simulink model "DYNctl_ver4_etud_obfusc"  (R2019a)
settings: Solver=ode45  StartTime=0.0  StopTime=tfin  FixedStep=0.001  RelTol=1e-09  EnableMultiTasking=on
values from neighbouring files (symbols this model uses):
  ae0 = 1.346257119209160    (= 1.34625711921)    [bancEssaiConstantes.m]
  ae1 = 3.490773781399032e+02    (= 349.07737814)    [bancEssaiConstantes.m]
  ae2 = 1.450384791542791e+03    (= 1450.38479154)    [bancEssaiConstantes.m]
  ae3 = 7.033442113266084e+05    (= 703344.211327)    [bancEssaiConstantes.m]
  as0 = 0.040978814093345    (= 0.0409788140933)    [bancEssaiConstantes.m]
  as1 = 10.275913216141866    (= 10.2759132161)    [bancEssaiConstantes.m]
  as2 = -4.149770657537117e+02    (= -414.977065754)    [bancEssaiConstantes.m]
  as3 = 5.763371762601417e+03    (= 5763.3717626)    [bancEssaiConstantes.m]
  be1 = 13.029359254409743    (= 13.0293592544)    [bancEssaiConstantes.m]
  g = 9.81    [bancEssaiConstantes.m]
  Jx = 1169e-06    (= 0.001169)    [bancEssaiConstantes.m]
  LL = .115    (= 0.115)    [bancEssaiConstantes.m]
  mP = 425e-03    (= 0.425)    [bancEssaiConstantes.m]
  mS = 0.0080    (= 0.008)    [bancEssaiConstantes.m]
  offset = 7.563899999998686    (= 7.5639)    [bancEssaiConstantes.m]
  RR = 3.6    [bancEssaiConstantes.m]
  Vmax = 16.0    (= 16)    [bancEssaiConstantes.m]
  XA = +rABC    (= 0.0952)    [bancEssaiConstantes.m]
  XB = -rABC*sind(30)    [bancEssaiConstantes.m]
  XC = -rABC*sind(30)    [bancEssaiConstantes.m]
  XD = +rDEF*sind(30)    [bancEssaiConstantes.m]
  XE = -rDEF    (= -0.08)    [bancEssaiConstantes.m]
  XF = +rDEF*sind(30)    [bancEssaiConstantes.m]
  YA = 0.0    (= 0)    [bancEssaiConstantes.m]
  YB = +rABC*cosd(30)    [bancEssaiConstantes.m]
  YC = -rABC*cosd(30)    [bancEssaiConstantes.m]
  YD = +rDEF*cosd(30)    [bancEssaiConstantes.m]
  YE = 0.0    (= 0)    [bancEssaiConstantes.m]
  YF = -rDEF*cosd(30)    [bancEssaiConstantes.m]
settings Model: Creator=delafontaine  LastModifiedBy=gaul2525
settings SolverCC: AlgebraicLoopSolver=LineSearch
settings DataIOCC: LimitDataPoints=on  SaveFormat=Array  SignalLoggingSaveFormat=ModelDataLogs  ReturnWorkspaceOutputs=off
settings OptimizationCC: LifeSpan=inf
settings DebuggingCC: UnderspecifiedInitializationDetection=Classic  MergeDetectMultiDrivingBlocksExec=none  MultiTaskDSMMsg=warning  MultiTaskCondExecSysMsg=none  SFUnexpectedBacktrackingDiag=warning  SFNoUnconditionalDefaultTransitionDiag=warning  SFExecutionAtInitializationDiag=none  UnderSpecifiedDimensionMsg=warning  ArithmeticOperatorsInVariantConditions=warning
settings HardwareCC: ProdBitPerPointer=32  ProdBitPerSizeT=32  ProdBitPerPtrDiffT=32  ProdLargestAtomicFloat=None  ProdIntDivRoundTo=Undefined  ProdEndianess=Unspecified  ProdWordSize=32  ProdHWDeviceType=32-bit Generic
settings ModelReferenceCC: PropagateSignalLabelsOutOfModel=off
settings SFSimCC: SimUseLocalCustomCode=off
settings RTWCC: RTWUseLocalCustomCode=off
settings CodeAppCC: StateflowObjectComments=on
settings GRTTargetCC: TargetLangStandard=C89/C90 (ANSI)  GeneratePreprocessorConditionals=Disable all
settings ConfigComp: CovMetricSettings=dw  CovHtmlReporting=on  CovSaveCumulativeToWorkspaceVar=on  CovSaveSingleToWorkspaceVar=on  CovExternalEMLEnable=off  CovSFcnEnable=off

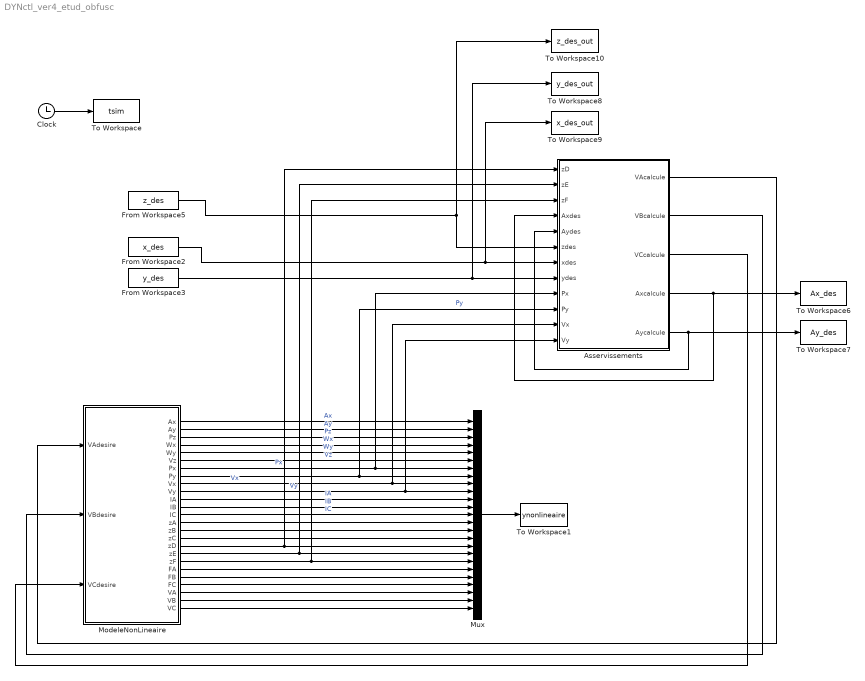
== system DYNctl_ver4_etud_obfusc ==
  Asservissements : Subsystem
      mask help: Simulink:masks:GenSFuncDesc_MD
      mask Help: eval('feval(''rtwprivate'',''rtwhelpview'',''rtw_sfcn_block'')');
  Clock : Clock
  From Workspace2 : FromWorkspace  VariableName=x_des  SampleTime=0  Interpolate=off  OutputAfterFinalValue=Holding final value
  From Workspace3 : FromWorkspace  VariableName=y_des  SampleTime=0  Interpolate=off  OutputAfterFinalValue=Holding final value
  From Workspace5 : FromWorkspace  VariableName=z_des  SampleTime=0  Interpolate=off  OutputAfterFinalValue=Holding final value
  ModeleNonLineaire : Subsystem
      mask help: Simulink:masks:GenSFuncDesc_MD
      mask Help: eval('feval(''rtwprivate'',''rtwhelpview'',''rtw_sfcn_block'')');
  Mux : Mux  Inputs=25
  To Workspace : ToWorkspace  VariableName=tsim  SampleTime=-1
  To Workspace1 : ToWorkspace  VariableName=ynonlineaire  SampleTime=-1
  To Workspace10 : ToWorkspace  VariableName=z_des_out  SampleTime=-1
  To Workspace6 : ToWorkspace  VariableName=Ax_des  SampleTime=-1
  To Workspace7 : ToWorkspace  VariableName=Ay_des  SampleTime=-1
  To Workspace8 : ToWorkspace  VariableName=y_des_out  SampleTime=-1
  To Workspace9 : ToWorkspace  VariableName=x_des_out  SampleTime=-1
  wires:
  Mux/1 -> To Workspace1/1
  Clock/1 -> To Workspace/1
  From Workspace5/1 -> Asservissements/6(zdes), To Workspace10/1
  ModeleNonLineaire/1(Ax) -> Mux/1  "Ax"
  ModeleNonLineaire/2(Ay) -> Mux/2  "Ay"
  ModeleNonLineaire/3(Pz) -> Mux/3  "Pz"
  ModeleNonLineaire/4(Wx) -> Mux/4  "Wx"
  ModeleNonLineaire/5(Wy) -> Mux/5  "Wy"
  ModeleNonLineaire/6(Vz) -> Mux/6  "Vz"
  ModeleNonLineaire/7(Px) -> Asservissements/9(Px), Mux/7  "Px"
  ModeleNonLineaire/8(Py) -> Asservissements/10(Py), Mux/8  "Py"
  ModeleNonLineaire/9(Vx) -> Asservissements/11(Vx), Mux/9  "Vx"
  ModeleNonLineaire/10(Vy) -> Asservissements/12(Vy), Mux/10  "Vy"
  ModeleNonLineaire/11(IA) -> Mux/11  "IA"
  ModeleNonLineaire/12(IB) -> Mux/12  "IB"
  ModeleNonLineaire/13(IC) -> Mux/13  "IC"
  From Workspace3/1 -> Asservissements/8(ydes), To Workspace8/1
  From Workspace2/1 -> Asservissements/7(xdes), To Workspace9/1
  ModeleNonLineaire/20(FA) -> Mux/20
  ModeleNonLineaire/21(FB) -> Mux/21
  ModeleNonLineaire/22(FC) -> Mux/22
  ModeleNonLineaire/23(VA) -> Mux/23
  ModeleNonLineaire/24(VB) -> Mux/24
  ModeleNonLineaire/25(VC) -> Mux/25
  ModeleNonLineaire/17(zD) -> Asservissements/1(zD), Mux/17
  ModeleNonLineaire/18(zE) -> Asservissements/2(zE), Mux/18
  ModeleNonLineaire/19(zF) -> Asservissements/3(zF), Mux/19
  ModeleNonLineaire/14(zA) -> Mux/14
  ModeleNonLineaire/15(zB) -> Mux/15
  ModeleNonLineaire/16(zC) -> Mux/16
  Asservissements/4(Axcalcule) -> Asservissements/4(Axdes), To Workspace6/1
  Asservissements/5(Aycalcule) -> Asservissements/5(Aydes), To Workspace7/1
  Asservissements/1(VAcalcule) -> ModeleNonLineaire/1(VAdesire)
  Asservissements/2(VBcalcule) -> ModeleNonLineaire/2(VBdesire)
  Asservissements/3(VCcalcule) -> ModeleNonLineaire/3(VCdesire)

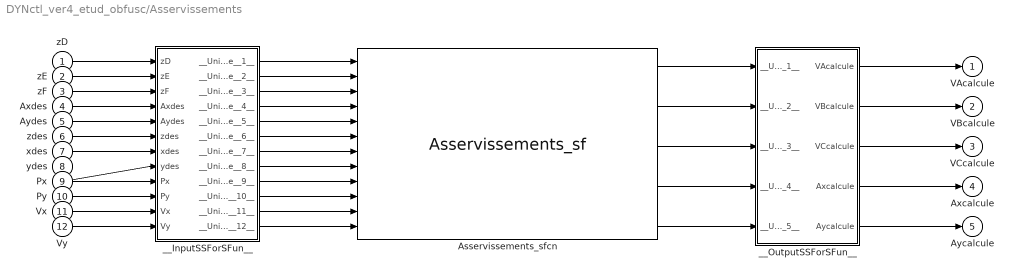
== system DYNctl_ver4_etud_obfusc/Asservissements ==
  zD : Inport
  zE : Inport  Port=2
  zF : Inport  Port=3
  Axdes : Inport  Port=4
  Aydes : Inport  Port=5
  zdes : Inport  Port=6
  xdes : Inport  Port=7
  ydes : Inport  Port=8
  Px : Inport  Port=9
  Py : Inport  Port=10
  Vx : Inport  Port=11
  Vy : Inport  Port=12
  Asservissements_sfcn : S-Function  FunctionName=Asservissements_sf  SFunctionModules=""  SFunctionDeploymentMode=off  EnableBusSupport=off  mask{rtw_sf_name=Asservissements_sf, showVar=off}
      mask prompts: rtw_sf_name "Simulink:masks:GenSFuncName_MP"; showVar "Simulink:masks:GenSFuncShowModuleList_MP"
      mask help: Simulink:masks:GenSFuncDesc_MD
      mask init:
      | displist = '';
      | if ~strcmp(get_param(gcb, 'FunctionName'), rtw_sf_name);
      |   set_param(gcb, 'FunctionName', rtw_sf_name);
      | end
      | % Check if we are generating code
      | rtw_mode = false;
      | if strcmpi(get_param(bdroot(gcb),'SimulationStatus'),'Initializing')
      | 	rtw_mode = strcmpi(get_param(bdroot(gcb),'BuildingRTWCode'),'on') && ...
      | 		~strcmpi(get_param(bdroot(gcb),'TargetStyle'),'SimulationTarget');
      | end
      | if showVar || rtw_mode
      | 	if exist('rtwsfunc') == 2 | exist('rtwsfunc') == 6
      | 		tmplist = rtwsfunc(rtw_sf_name,gcb);
      | 		tmplist = DAStudio.message('Simulink:masks:GenSFuncListOfModules_IC', tmplist);
      | 	elseif showVar
      | 		tmplist1 = DAStudio.message('Simulink:masks:GenSFuncListOfModules_IC', '');
      |         tmplist2 = DAStudio.message('Simulink:masks:GenSFuncNotLicensed_IC');
      |         tmplist = [tmplist1 tmplist2];
      |  	end
      | end
      | if showVar
      |   displist = tmplist;
      | end
      settings: CopyFcn=|
      | if ~strcmp(get_param(gcb,'Linkstatus'),'none') && ...
      | ~strcmp(get_param(gcb,'Linkstatus'),'implicit')
      |   set_param(gcb,'LinkStatus','none');
      | end
      mask Help: eval('feval(''rtwprivate'',''rtwhelpview'',''rtw_sfcn_block'')');
      mask Display:
      | port_label('input',1,'zD');
      | port_label('input',2,'zE');
      | port_label('input',3,'zF');
      | port_label('input',4,'Axdes');
      | port_label('input',5,'Aydes');
      | port_label('input',6,'zdes');
      | port_label('input',7,'xdes');
      | port_label('input',8,'ydes');
      | port_label('input',9,'Px');
      | port_label('input',10,'Py');
      | port_label('input',11,'Vx');
      | port_label('input',12,'Vy');
      | port_label('output',1,'VAcalcule');
      | port_label('output',2,'VBcalcule');
      | port_label('output',3,'VCcalcule');
      | port_label('output',4,'Axcalcule');
      | port_label('output',5,'Aycalcule');
  __InputSSForSFun__ : Subsystem
  __OutputSSForSFun__ : Subsystem
  VAcalcule : Outport
  VBcalcule : Outport  Port=2
  VCcalcule : Outport  Port=3
  Axcalcule : Outport  Port=4
  Aycalcule : Outport  Port=5
  wires:
  zD/1 -> __InputSSForSFun__/1(zD)
  zE/1 -> __InputSSForSFun__/2(zE)
  zF/1 -> __InputSSForSFun__/3(zF)
  Axdes/1 -> __InputSSForSFun__/4(Axdes)
  Aydes/1 -> __InputSSForSFun__/5(Aydes)
  zdes/1 -> __InputSSForSFun__/6(zdes)
  xdes/1 -> __InputSSForSFun__/7(xdes)
  ydes/1 -> __InputSSForSFun__/8(ydes)
  Px/1 -> __InputSSForSFun__/9(Px)
  Py/1 -> __InputSSForSFun__/10(Py)
  Vx/1 -> __InputSSForSFun__/11(Vx)
  Vy/1 -> __InputSSForSFun__/12(Vy)
  __InputSSForSFun__/1(__UniqueOutportName__1__) -> Asservissements_sfcn/1
  __InputSSForSFun__/2(__UniqueOutportName__2__) -> Asservissements_sfcn/2
  __InputSSForSFun__/3(__UniqueOutportName__3__) -> Asservissements_sfcn/3
  __InputSSForSFun__/4(__UniqueOutportName__4__) -> Asservissements_sfcn/4
  __InputSSForSFun__/5(__UniqueOutportName__5__) -> Asservissements_sfcn/5
  __InputSSForSFun__/6(__UniqueOutportName__6__) -> Asservissements_sfcn/6
  __InputSSForSFun__/7(__UniqueOutportName__7__) -> Asservissements_sfcn/7
  __InputSSForSFun__/8(__UniqueOutportName__8__) -> Asservissements_sfcn/8
  __InputSSForSFun__/9(__UniqueOutportName__9__) -> Asservissements_sfcn/9
  __InputSSForSFun__/10(__UniqueOutportName__10__) -> Asservissements_sfcn/10
  __InputSSForSFun__/11(__UniqueOutportName__11__) -> Asservissements_sfcn/11
  __InputSSForSFun__/12(__UniqueOutportName__12__) -> Asservissements_sfcn/12
  Asservissements_sfcn/1 -> __OutputSSForSFun__/1(__UniqueInportName__1__)
  Asservissements_sfcn/2 -> __OutputSSForSFun__/2(__UniqueInportName__2__)
  Asservissements_sfcn/3 -> __OutputSSForSFun__/3(__UniqueInportName__3__)
  Asservissements_sfcn/4 -> __OutputSSForSFun__/4(__UniqueInportName__4__)
  Asservissements_sfcn/5 -> __OutputSSForSFun__/5(__UniqueInportName__5__)
  __OutputSSForSFun__/1(VAcalcule) -> VAcalcule/1
  __OutputSSForSFun__/2(VBcalcule) -> VBcalcule/1
  __OutputSSForSFun__/3(VCcalcule) -> VCcalcule/1
  __OutputSSForSFun__/4(Axcalcule) -> Axcalcule/1
  __OutputSSForSFun__/5(Aycalcule) -> Aycalcule/1

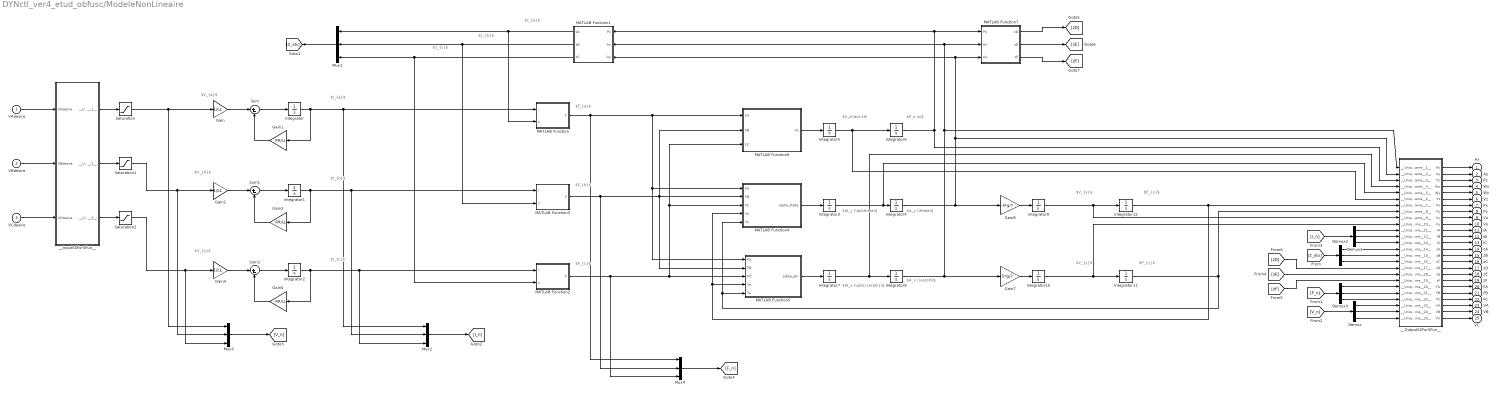
== system DYNctl_ver4_etud_obfusc/ModeleNonLineaire ==
  note: $z_{c}$
  note: $V_{x}$
  note: $I_{a}$
  note: $P_{x}$
  note: $I_{c}$
  note: $z_{b}$
  note: $F_{a}$
  note: $V_{y}$
  note: $V_{b}$
  note: $F_{b}$
  note: $F_{c}$
  note: $P_{y}$
  note: $V_{c}$
  note: $V_z(\dot z)$
  note: $z_{a}$
  note: $I_{b}$
  note: $V_{a}$
  note: $A_y (\theta)$
  note: $A_x (\varphi)$
  note: $W_x (\dot{\varphi})$
  note: $W_y (\dot\theta)$
  note: $P_z (z)$
  VAdesire : Inport
  VBdesire : Inport  Port=2
  VCdesire : Inport  Port=3
  Demux{,1..3} (4 alike) : Demux  Outputs=3
  Gain : Gain  Gain=1/LL
  Gain1 : Gain  Gain=RR/LL
  Gain2 : Gain  Gain=1/LL
  Gain3 : Gain  Gain=RR/LL
  Gain4 : Gain  Gain=1/LL
  Gain5 : Gain  Gain=RR/LL
  Gain7 : Gain  Gain=5*g/7
  Gain8 : Gain  Gain=-5*g/7
  Integrator : Integrator  InitialCondition=-0.4961
  Integrator1 : Integrator  InitialCondition=-0.4961
  Integrator{3..5,7..12} (9 alike) : Integrator
  Integrator2 : Integrator  InitialCondition=-0.4961
  Integrator6 : Integrator  InitialCondition=0.015
  MATLAB Function : MATLAB Function  TreatAsAtomicUnit=on
  MATLAB Function1 : MATLAB Function  TreatAsAtomicUnit=on
  MATLAB Function2 : MATLAB Function  TreatAsAtomicUnit=on
  MATLAB Function3 : MATLAB Function  TreatAsAtomicUnit=on
  MATLAB Function4 : MATLAB Function  TreatAsAtomicUnit=on
  MATLAB Function5 : MATLAB Function  TreatAsAtomicUnit=on
  MATLAB Function6 : MATLAB Function  TreatAsAtomicUnit=on
  MATLAB Function7 : MATLAB Function  TreatAsAtomicUnit=on
  Mux{1..4} (4 alike) : Mux  Inputs=3
  Saturation : Saturate  UpperLimit=Vmax  LowerLimit=-Vmax
  Saturation1 : Saturate  UpperLimit=Vmax  LowerLimit=-Vmax
  Saturation2 : Saturate  UpperLimit=Vmax  LowerLimit=-Vmax
  Sum : Sum  Inputs=|+-
  Sum1 : Sum  Inputs=|+-
  Sum2 : Sum  Inputs=|+-
  __InputSSForSFun__ : Subsystem
  __OutputSSForSFun__ : Subsystem
  Ax : Outport
  Ay : Outport  Port=2
  Pz : Outport  Port=3
  Wx : Outport  Port=4
  Wy : Outport  Port=5
  Vz : Outport  Port=6
  Px : Outport  Port=7
  Py : Outport  Port=8
  Vx : Outport  Port=9
  Vy : Outport  Port=10
  IA : Outport  Port=11
  IB : Outport  Port=12
  IC : Outport  Port=13
  zA : Outport  Port=14
  zB : Outport  Port=15
  zC : Outport  Port=16
  zD : Outport  Port=17
  zE : Outport  Port=18
  zF : Outport  Port=19
  FA : Outport  Port=20
  FB : Outport  Port=21
  FC : Outport  Port=22
  VA : Outport  Port=23
  VB : Outport  Port=24
  VC : Outport  Port=25
  wires:
  VAdesire/1 -> __InputSSForSFun__/1(VAdesire)
  VBdesire/1 -> __InputSSForSFun__/2(VBdesire)
  VCdesire/1 -> __InputSSForSFun__/3(VCdesire)
  __InputSSForSFun__/1(__UniqueOutportName__1__) -> Saturation/1
  __InputSSForSFun__/2(__UniqueOutportName__2__) -> Saturation1/1
  __InputSSForSFun__/3(__UniqueOutportName__3__) -> Saturation2/1
  __OutputSSForSFun__/1(Ax) -> Ax/1
  __OutputSSForSFun__/2(Ay) -> Ay/1
  __OutputSSForSFun__/3(Pz) -> Pz/1
  __OutputSSForSFun__/4(Wx) -> Wx/1
  __OutputSSForSFun__/5(Wy) -> Wy/1
  __OutputSSForSFun__/6(Vz) -> Vz/1
  __OutputSSForSFun__/7(Px) -> Px/1
  __OutputSSForSFun__/8(Py) -> Py/1
  __OutputSSForSFun__/9(Vx) -> Vx/1
  __OutputSSForSFun__/10(Vy) -> Vy/1
  __OutputSSForSFun__/11(IA) -> IA/1
  __OutputSSForSFun__/12(IB) -> IB/1
  __OutputSSForSFun__/13(IC) -> IC/1
  __OutputSSForSFun__/14(zA) -> zA/1
  __OutputSSForSFun__/15(zB) -> zB/1
  __OutputSSForSFun__/16(zC) -> zC/1
  __OutputSSForSFun__/17(zD) -> zD/1
  __OutputSSForSFun__/18(zE) -> zE/1
  __OutputSSForSFun__/19(zF) -> zF/1
  __OutputSSForSFun__/20(FA) -> FA/1
  __OutputSSForSFun__/21(FB) -> FB/1
  __OutputSSForSFun__/22(FC) -> FC/1
  __OutputSSForSFun__/23(VA) -> VA/1
  __OutputSSForSFun__/24(VB) -> VB/1
  __OutputSSForSFun__/25(VC) -> VC/1
  Sum2/1 -> Integrator2/1
  Integrator/1 -> MATLAB Function/1(i), Mux2/1, Gain1/1
  Integrator8/1 -> Gain7/1, __OutputSSForSFun__/1(__UniqueInportName__1__), MATLAB Function1/2(Ax), MATLAB Function7/2(Ax)
  Integrator1/1 -> MATLAB Function3/1(i), Mux2/2, Gain3/1
  MATLAB Function1/3(zC) -> MATLAB Function2/2(z), Mux1/3
  MATLAB Function/1(F) -> Mux4/1, MATLAB Function6/1(FA), MATLAB Function4/1(FA), MATLAB Function5/1(FA)
  Sum1/1 -> Integrator1/1
  MATLAB Function5/1(alpha_phi) -> Integrator7/1
  MATLAB Function6/1(Az) -> Integrator5/1
  Sum/1 -> Integrator/1
  Gain3/1 -> Sum1/2
  Integrator2/1 -> Gain5/1, MATLAB Function2/1(i), Mux2/3
  Integrator7/1 -> Integrator8/1, __OutputSSForSFun__/4(__UniqueInportName__4__)
  Gain5/1 -> Sum2/2
  MATLAB Function1/1(zA) -> MATLAB Function/2(z), Mux1/1
  Integrator12/1 -> __OutputSSForSFun__/7(__UniqueInportName__7__), MATLAB Function5/4(Xs), MATLAB Function4/4(Xs)
  Gain7/1 -> Integrator10/1
  Integrator11/1 -> __OutputSSForSFun__/8(__UniqueInportName__8__), MATLAB Function4/5(Ys), MATLAB Function5/5(Ys)
  Integrator6/1 -> MATLAB Function1/1(Pz), MATLAB Function7/1(Pz), __OutputSSForSFun__/3(__UniqueInportName__3__)
  Gain8/1 -> Integrator9/1
  Integrator3/1 -> __OutputSSForSFun__/5(__UniqueInportName__5__), Integrator4/1
  Integrator9/1 -> Integrator12/1, __OutputSSForSFun__/9(__UniqueInportName__9__)
  Gain2/1 -> Sum1/1
  Integrator10/1 -> Integrator11/1, __OutputSSForSFun__/10(__UniqueInportName__10__)
  Integrator4/1 -> Gain8/1, MATLAB Function1/3(Ay), MATLAB Function7/3(Ay), __OutputSSForSFun__/2(__UniqueInportName__2__)
  MATLAB Function4/1(alpha_theta) -> Integrator3/1
  MATLAB Function2/1(F) -> Mux4/3, MATLAB Function5/3(FC), MATLAB Function4/3(FC), MATLAB Function6/3(FC)
  Gain/1 -> Sum/1
  Gain4/1 -> Sum2/1
  MATLAB Function3/1(F) -> Mux4/2, MATLAB Function4/2(FB), MATLAB Function6/2(FB), MATLAB Function5/2(FB)
  Gain1/1 -> Sum/2
  MATLAB Function1/2(zB) -> MATLAB Function3/2(z), Mux1/2
  Integrator5/1 -> Integrator6/1, __OutputSSForSFun__/6(__UniqueInportName__6__)
  Mux1/1 -> [Z_abc]
  Mux2/1 -> [I_n]
  Mux3/1 -> [V_n]
  Demux/1 -> __OutputSSForSFun__/23(__UniqueInportName__23__)
  Demux/2 -> __OutputSSForSFun__/24(__UniqueInportName__24__)
  Demux/3 -> __OutputSSForSFun__/25(__UniqueInportName__25__)
  [V_n] -> Demux/1
  Demux1/1 -> __OutputSSForSFun__/11(__UniqueInportName__11__)
  Demux1/2 -> __OutputSSForSFun__/12(__UniqueInportName__12__)
  Demux1/3 -> __OutputSSForSFun__/13(__UniqueInportName__13__)
  [I_n] -> Demux1/1
  Demux2/1 -> __OutputSSForSFun__/14(__UniqueInportName__14__)
  Demux2/2 -> __OutputSSForSFun__/15(__UniqueInportName__15__)
  Demux2/3 -> __OutputSSForSFun__/16(__UniqueInportName__16__)
  [Z_abc] -> Demux2/1
  Mux4/1 -> [F_n]
  [F_n] -> Demux3/1
  Demux3/3 -> __OutputSSForSFun__/22(__UniqueInportName__22__)
  Demux3/2 -> __OutputSSForSFun__/21(__UniqueInportName__21__)
  Demux3/1 -> __OutputSSForSFun__/20(__UniqueInportName__20__)
  [zD] -> __OutputSSForSFun__/17(__UniqueInportName__17__)
  [zE] -> __OutputSSForSFun__/18(__UniqueInportName__18__)
  [zF] -> __OutputSSForSFun__/19(__UniqueInportName__19__)
  MATLAB Function7/1(zD) -> [zD]
  MATLAB Function7/2(zE) -> [zE]
  MATLAB Function7/3(zF) -> [zF]
  Saturation/1 -> Gain/1, Mux3/1
  Saturation1/1 -> Mux3/2, Gain2/1
  Saturation2/1 -> Mux3/3, Gain4/1

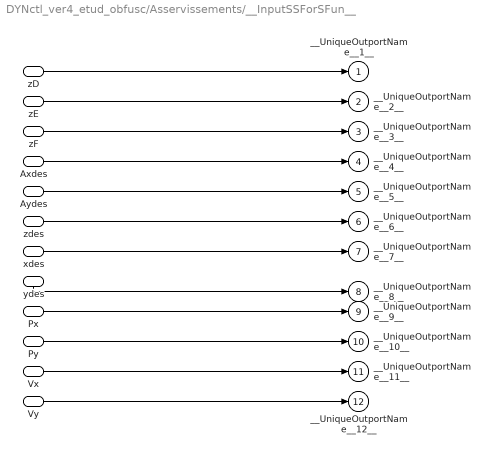
== system DYNctl_ver4_etud_obfusc/Asservissements/__InputSSForSFun__ ==
  zD : Inport
  zE : Inport  Port=2
  zF : Inport  Port=3
  Axdes : Inport  Port=4
  Aydes : Inport  Port=5
  zdes : Inport  Port=6
  xdes : Inport  Port=7
  ydes : Inport  Port=8
  Px : Inport  Port=9
  Py : Inport  Port=10
  Vx : Inport  Port=11
  Vy : Inport  Port=12
  __UniqueOutportName__1__ : Outport
  __UniqueOutportName__2__ : Outport  Port=2
  __UniqueOutportName__3__ : Outport  Port=3
  __UniqueOutportName__4__ : Outport  Port=4
  __UniqueOutportName__5__ : Outport  Port=5
  __UniqueOutportName__6__ : Outport  Port=6
  __UniqueOutportName__7__ : Outport  Port=7
  __UniqueOutportName__8__ : Outport  Port=8
  __UniqueOutportName__9__ : Outport  Port=9
  __UniqueOutportName__10__ : Outport  Port=10
  __UniqueOutportName__11__ : Outport  Port=11
  __UniqueOutportName__12__ : Outport  Port=12
  wires:
  zD/1 -> __UniqueOutportName__1__/1
  zE/1 -> __UniqueOutportName__2__/1
  zF/1 -> __UniqueOutportName__3__/1
  Axdes/1 -> __UniqueOutportName__4__/1
  Aydes/1 -> __UniqueOutportName__5__/1
  zdes/1 -> __UniqueOutportName__6__/1
  xdes/1 -> __UniqueOutportName__7__/1
  ydes/1 -> __UniqueOutportName__8__/1
  Px/1 -> __UniqueOutportName__9__/1
  Py/1 -> __UniqueOutportName__10__/1
  Vx/1 -> __UniqueOutportName__11__/1
  Vy/1 -> __UniqueOutportName__12__/1

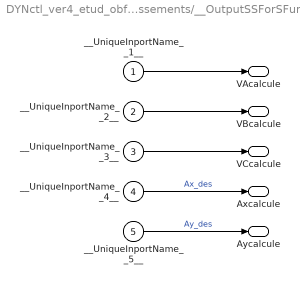
== system DYNctl_ver4_etud_obfusc/Asservissements/__OutputSSForSFun__ ==
  __UniqueInportName__1__ : Inport
  __UniqueInportName__2__ : Inport  Port=2
  __UniqueInportName__3__ : Inport  Port=3
  __UniqueInportName__4__ : Inport  Port=4
  __UniqueInportName__5__ : Inport  Port=5
  VAcalcule : Outport
  VBcalcule : Outport  Port=2
  VCcalcule : Outport  Port=3
  Axcalcule : Outport  Port=4
  Aycalcule : Outport  Port=5
  wires:
  __UniqueInportName__1__/1 -> VAcalcule/1
  __UniqueInportName__2__/1 -> VBcalcule/1
  __UniqueInportName__3__/1 -> VCcalcule/1
  __UniqueInportName__4__/1 -> Axcalcule/1  "Ax_des"
  __UniqueInportName__5__/1 -> Aycalcule/1  "Ay_des"

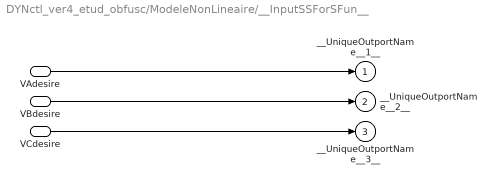
== system DYNctl_ver4_etud_obfusc/ModeleNonLineaire/__InputSSForSFun__ ==
  VAdesire : Inport
  VBdesire : Inport  Port=2
  VCdesire : Inport  Port=3
  __UniqueOutportName__1__ : Outport
  __UniqueOutportName__2__ : Outport  Port=2
  __UniqueOutportName__3__ : Outport  Port=3
  wires:
  VAdesire/1 -> __UniqueOutportName__1__/1
  VBdesire/1 -> __UniqueOutportName__2__/1
  VCdesire/1 -> __UniqueOutportName__3__/1

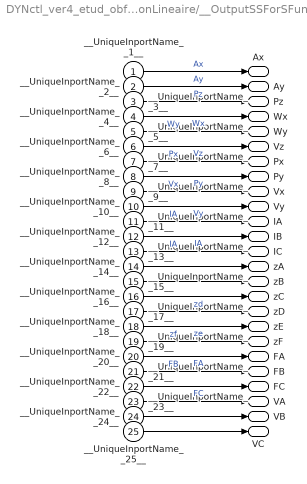
== system DYNctl_ver4_etud_obfusc/ModeleNonLineaire/__OutputSSForSFun__ ==
  __UniqueInportName__1__ : Inport
  __UniqueInportName__2__ : Inport  Port=2
  __UniqueInportName__3__ : Inport  Port=3
  __UniqueInportName__4__ : Inport  Port=4
  __UniqueInportName__5__ : Inport  Port=5
  __UniqueInportName__6__ : Inport  Port=6
  __UniqueInportName__7__ : Inport  Port=7
  __UniqueInportName__8__ : Inport  Port=8
  __UniqueInportName__9__ : Inport  Port=9
  __UniqueInportName__10__ : Inport  Port=10
  __UniqueInportName__11__ : Inport  Port=11
  __UniqueInportName__12__ : Inport  Port=12
  __UniqueInportName__13__ : Inport  Port=13
  __UniqueInportName__14__ : Inport  Port=14
  __UniqueInportName__15__ : Inport  Port=15
  __UniqueInportName__16__ : Inport  Port=16
  __UniqueInportName__17__ : Inport  Port=17
  __UniqueInportName__18__ : Inport  Port=18
  __UniqueInportName__19__ : Inport  Port=19
  __UniqueInportName__20__ : Inport  Port=20
  __UniqueInportName__21__ : Inport  Port=21
  __UniqueInportName__22__ : Inport  Port=22
  __UniqueInportName__23__ : Inport  Port=23
  __UniqueInportName__24__ : Inport  Port=24
  __UniqueInportName__25__ : Inport  Port=25
  Ax : Outport
  Ay : Outport  Port=2
  Pz : Outport  Port=3
  Wx : Outport  Port=4
  Wy : Outport  Port=5
  Vz : Outport  Port=6
  Px : Outport  Port=7
  Py : Outport  Port=8
  Vx : Outport  Port=9
  Vy : Outport  Port=10
  IA : Outport  Port=11
  IB : Outport  Port=12
  IC : Outport  Port=13
  zA : Outport  Port=14
  zB : Outport  Port=15
  zC : Outport  Port=16
  zD : Outport  Port=17
  zE : Outport  Port=18
  zF : Outport  Port=19
  FA : Outport  Port=20
  FB : Outport  Port=21
  FC : Outport  Port=22
  VA : Outport  Port=23
  VB : Outport  Port=24
  VC : Outport  Port=25
  wires:
  __UniqueInportName__1__/1 -> Ax/1  "Ax"
  __UniqueInportName__2__/1 -> Ay/1  "Ay"
  __UniqueInportName__3__/1 -> Pz/1  "Pz"
  __UniqueInportName__4__/1 -> Wx/1  "Wx"
  __UniqueInportName__5__/1 -> Wy/1  "Wy"
  __UniqueInportName__6__/1 -> Vz/1  "Vz"
  __UniqueInportName__7__/1 -> Px/1  "Px"
  __UniqueInportName__8__/1 -> Py/1  "Py"
  __UniqueInportName__9__/1 -> Vx/1  "Vx"
  __UniqueInportName__10__/1 -> Vy/1  "Vy"
  __UniqueInportName__11__/1 -> IA/1  "IA"
  __UniqueInportName__12__/1 -> IB/1  "IA"
  __UniqueInportName__13__/1 -> IC/1  "IA"
  __UniqueInportName__14__/1 -> zA/1
  __UniqueInportName__15__/1 -> zB/1
  __UniqueInportName__16__/1 -> zC/1
  __UniqueInportName__17__/1 -> zD/1  "zd"
  __UniqueInportName__18__/1 -> zE/1  "ze"
  __UniqueInportName__19__/1 -> zF/1  "zf"
  __UniqueInportName__20__/1 -> FA/1  "FA"
  __UniqueInportName__21__/1 -> FB/1  "FB"
  __UniqueInportName__22__/1 -> FC/1  "FC"
  __UniqueInportName__23__/1 -> VA/1
  __UniqueInportName__24__/1 -> VB/1
  __UniqueInportName__25__/1 -> VC/1

== matlab function DYNctl_ver4_etud_obfusc/ModeleNonLineaire/MATLAB Function1 ==
  data: Pz input; Ax input; zA output double size=1; Ay input; zB output double size=1; zC output double size=1; XA parameter size=1; XB parameter size=1; XC parameter size=1; YA parameter size=1; YB parameter size=1; YC parameter size=1
function [zA,zB,zC] = fcn(Pz, Ax , Ay, XA, XB, XC, YA, YB, YC)

    zA = Pz- XA*Ay + YA*Ax;
    
    zB = Pz- XB*Ay + YB*Ax;
    
    zC = Pz- XC*Ay + YC*Ax;

== matlab function DYNctl_ver4_etud_obfusc/ModeleNonLineaire/MATLAB Function ==
  data: i input size=1; F output double size=1; z input size=1; as0 parameter size=1; as1 parameter size=1; as2 parameter size=1; as3 parameter size=1; ae0 parameter size=1; ae1 parameter size=1; ae2 parameter size=1; ae3 parameter size=1; be1 parameter size=1; offset parameter size=1
function F = fcn(i , z, as0, as1, as2, as3, ae0, ae1, ae2, ae3, be1, offset)

    FSK = offset-1/(as0 + as1*z + as2*z^2 +as3*z^3);
    
    FEK = ((i^2 + be1*abs(i))*sign(i))/(ae0 + ae1*z + ae2*z^2 +ae3*z^3);

    F = FEK + FSK;

== matlab function DYNctl_ver4_etud_obfusc/ModeleNonLineaire/MATLAB Function2 ==
  data: i input size=1; F output double size=1; z input size=1; as0 parameter size=1; as1 parameter size=1; as2 parameter size=1; as3 parameter size=1; ae0 parameter size=1; ae1 parameter size=1; ae2 parameter size=1; ae3 parameter size=1; be1 parameter size=1; offset parameter size=1
function F = fcn(i , z, as0, as1, as2, as3, ae0, ae1, ae2, ae3, be1, offset)

    FSK = offset-1/(as0 + as1*z + as2*z^2 +as3*z^3);
    
    FEK = ((i^2 + be1*abs(i))*sign(i))/(ae0 + ae1*z + ae2*z^2 +ae3*z^3);

    F = FEK + FSK;

== matlab function DYNctl_ver4_etud_obfusc/ModeleNonLineaire/MATLAB Function3 ==
  data: i input size=1; F output double size=1; z input size=1; as0 parameter size=1; as1 parameter size=1; as2 parameter size=1; as3 parameter size=1; ae0 parameter size=1; ae1 parameter size=1; ae2 parameter size=1; ae3 parameter size=1; be1 parameter size=1; offset parameter size=1
function F = fcn(i , z, as0, as1, as2, as3, ae0, ae1, ae2, ae3, be1, offset)

    FSK = offset-1/(as0 + as1*z + as2*z^2 +as3*z^3);
    
    FEK = ((i^2 + be1*abs(i))*sign(i))/(ae0 + ae1*z + ae2*z^2 +ae3*z^3);

    F = FEK + FSK;

== matlab function DYNctl_ver4_etud_obfusc/ModeleNonLineaire/MATLAB Function4 ==
  data: FA input; alpha_theta output double size=1; FB input; FC input; Xs input; Ys input; Jx parameter size=1; mS parameter size=1; mP parameter size=1; g parameter size=1; XA parameter size=1; XB parameter size=1; XC parameter size=1
function alpha_theta = fcn(FA , FB , FC, Xs , Ys, Jx, mS, mP, g, XA, XB, XC)
    %Ay
    alpha_theta = (1/Jx)*(-FA*XA - FB*XB - FC*XC - Xs*mS*g);

== matlab function DYNctl_ver4_etud_obfusc/ModeleNonLineaire/MATLAB Function5 ==
  data: FA input; alpha_phi output double size=1; FB input; FC input; Xs input; Ys input; mS parameter size=1; mP parameter size=1; g parameter size=1; Jx parameter size=1; YA parameter size=1; YB parameter size=1; YC parameter size=1
function alpha_phi = fcn(FA , FB , FC, Xs , Ys, mS, mP, g, Jx, YA, YB, YC)

    alpha_phi = (1/Jx)*(FA*YA + FB*YB + FC*YC + mS*g*Ys);

== matlab function DYNctl_ver4_etud_obfusc/ModeleNonLineaire/MATLAB Function6 ==
  data: FA input; Az output double size=1; FB input; FC input; mS parameter size=1; mP parameter size=1; g parameter size=1
function Az = fcn(FA , FB , FC, mS, mP, g)

    Az = (FA + FB + FC + mS*g + mP*g)/mP;

== matlab function DYNctl_ver4_etud_obfusc/ModeleNonLineaire/MATLAB Function7 ==
  data: Pz input size=1; Ax input size=1; zD output double size=1; Ay input size=1; zE output double size=1; zF output double size=1; XD parameter size=1; YD parameter size=1; XE parameter size=1; YE parameter size=1; XF parameter size=1; YF parameter size=1
function [zD,zE,zF] = fcn(Pz , Ax , Ay, XD, YD, XE, YE, XF, YF)

    zD = Pz- XD*Ay + YD*Ax;
    
    zE = Pz- XE*Ay + YE*Ax;
    
    zF = Pz- XF*Ay + YF*Ax;
